simulink model "PMSM_lab"  (Simulink 10.0)
settings: Solver=ode4  StartTime=0.0  StopTime=2  FixedStep=1e-4  RelTol=1e-3  EnableMultiTasking=on
InitFcn:
  | Vdc=530;
  | P=8;
  | Rs=1.477;
  | Lds=19.75e-3;
  | Lqs=22.5e-3;
  | flux=0.2068;
  | J=0.0015806;
  | B=0.0034;
  | Wc=2*pi*500;
  | PM=75*pi/180;
  | Wc_kp_by_kids=tan(PM-pi/2+atan(Wc*Lds/Rs));
  | kids=Wc*sqrt(Rs*Rs+(Wc*Lds)^2)/sqrt(Wc_kp_by_kids^2+1);
  | kpds=Wc_kp_by_kids*kids/Wc;
  | Wc_kp_by_kiqs=tan(PM-pi/2+atan(Wc*Lqs/Rs));
  | kiqs=Wc*sqrt(Rs*Rs+(Wc*Lqs)^2)/sqrt(Wc_kp_by_kiqs^2+1);
  | kpqs=Wc_kp_by_kiqs*kiqs/Wc;
  | Wcw=2*pi*42;
  | PM=78*pi/180;
  | Wc_kp_by_kiw=tan(PM-pi/2+atan(Wcw*J/B));
  | kiw=(Wcw*sqrt(B*B+(Wcw*J)^2))/((3/2)*(P/2)*flux*sqrt(Wc_kp_by_kiw^2+1));
  | kpw=Wc_kp_by_kiw*kiw/Wcw;
  | 
  | 
  | PM  = 75;
  | Wc = 3140;
  | R=1.6;
  | Lq = 0.0225;
  | Ld = 0.01975;
  | 
  | PI_q = tand(PM - 90 + atand((Wc*Lq)/R));
  | Ki_q = (Wc * sqrt(((R)^2)+((Wc*Lq)^2))/sqrt(1+(PI_q)^2));
  | Kp_q = (PI_q * Ki_q)/Wc;
  | PI_d = tand(PM - 90 + atand((Wc*Ld)/R));
  | Ki_d = (Wc * sqrt(((R)^2)+((Wc*Ld)^2))/sqrt(1+(PI_d)^2));
  | Kp_d = (PI_d * Ki_d)/Wc;
  | 
  | 
  | Wc=2*pi*42;
  | PM=78;
  | wpi=tand(PM-90+atand((Wc*180/pi)*J/B));
  | Ki= (Wc * sqrt(B^2 + (Wc*J)^2))/(sqrt(1+(wpi)^2));
  | Kp= (wpi*Ki)/(Wc);
libraries: simulink x4, dsparch4 x3
settings Model: Creator=Gopi  LastModifiedBy=kanth
settings DataIOCC: LimitDataPoints=on  SignalLoggingSaveFormat=ModelDataLogs
settings OptimizationCC: ExpressionDepthLimit=2147483647
settings DebuggingCC: SolverPrmCheckMsg=warning  FcnCallInpInsideContextMsg=warning  StateNameClashWarn=warning
settings SFSimCC: SimParseCustomCode=off
settings GRTTargetCC: GeneratePreprocessorConditionals=Disable all
settings ConfigComp: CovExternalEMLEnable=off

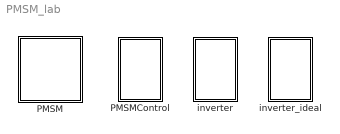
== system PMSM_lab ==
  PMSM : Subsystem
  PMSMControl : Subsystem
  inverter : Subsystem
  inverter_ideal : Subsystem

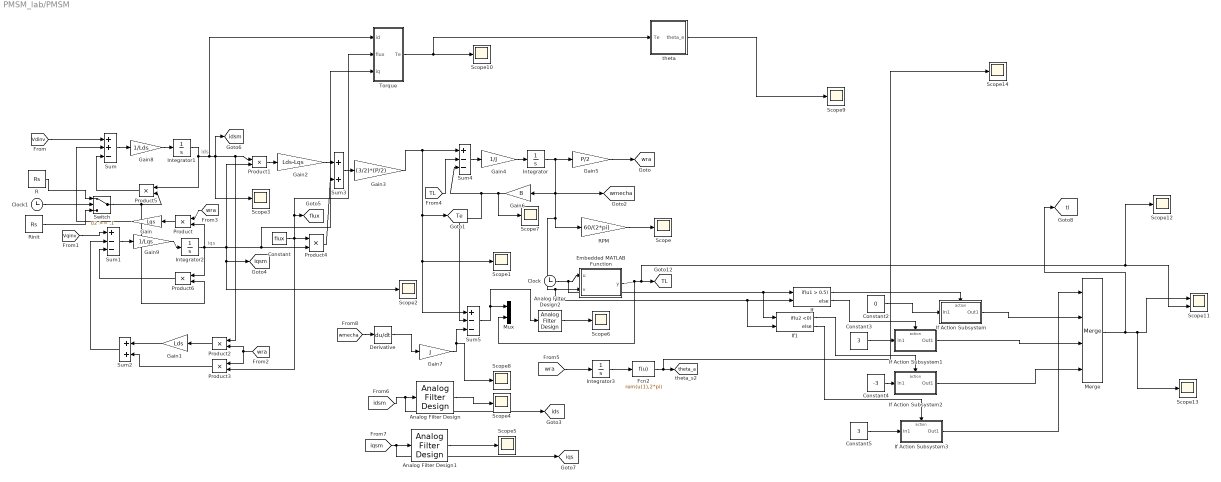
== system PMSM_lab/PMSM ==
  note: ids
  note: iqs
  Analog Filter Design : dsparch4/Analog Filter Design  method=Butterworth  filttype=Lowpass  N=1  Wlo=2*pi*1200  Whi=80  Rp=2  Rs=40
  Analog Filter Design1 : dsparch4/Analog Filter Design  method=Butterworth  filttype=Lowpass  N=1  Wlo=2*pi*800  Whi=80  Rp=2  Rs=40
  Analog Filter Design2 : dsparch4/Analog Filter Design  method=Butterworth  filttype=Lowpass  N=2  Wlo=2*pi*1000  Whi=80  Rp=2  Rs=40
  Clock : Clock
  Clock1 : Clock
  Constant : Constant  Value=flux
  Constant2 : Constant  Value=0
  Constant3 : Constant  Value=3
  Constant4 : Constant  Value=-3
  Constant5 : Constant  Value=3
  Derivative : Derivative
  Embedded MATLAB Function : MATLAB Function  TreatAsAtomicUnit=on
  Fcn2 : Fcn  Expr=rem(u(1),2*pi)
  Gain : Gain  Gain=Lqs
  Gain1 : Gain  Gain=Lds
  Gain2 : Gain  Gain=Lds-Lqs
  Gain3 : Gain  Gain=(3/2)*(P/2)
  Gain4 : Gain  Gain=1/J
  Gain5 : Gain  Gain=P/2
  Gain6 : Gain  Gain=B
  Gain7 : Gain  Gain=J
  Gain8 : Gain  Gain=1/Lds
  Gain9 : Gain  Gain=1/Lqs
  If : If  NumInputs=2  IfExpression=u1 > 0.5
  If Action Subsystem : Subsystem  TreatAsAtomicUnit=on
  If Action Subsystem1 : Subsystem  TreatAsAtomicUnit=on
  If Action Subsystem2 : Subsystem  TreatAsAtomicUnit=on
  If Action Subsystem3 : Subsystem  TreatAsAtomicUnit=on
  If1 : If  NumInputs=2  IfExpression=u2 <0
  Integrator{,1..3} (4 alike) : Integrator
  Merge : Merge  Inputs=4
  Mux : Mux  Inputs=2
  Product{,1..6} (7 alike) : Product  RndMeth=Zero
  R : Constant  Value=Rs
  RPM : Gain  Gain=60/(2*pi)
  Rinit : Constant  Value=Rs
  Scope{,1..10,12..14} (14 alike) : Scope
  Scope11 : Scope  NumInputPorts=2
  Sum : Sum  Inputs=++-
  Sum1 : Sum  Inputs=+--
  Sum2 : Sum
  Sum3 : Sum
  Sum4 : Sum  Inputs=+--
  Sum5 : Sum  Inputs=+--
  Switch : Switch  Threshold=.1
  Torque : Subsystem
  theta : Subsystem
  tag scope: TL=global, Te=global, flux=global, ids=global, idsm=global, iqs=global, iqsm=global, theta_a=global, tl=global, wmecha=global, wra=global
  wires:
  [Vdinv] -> Sum/1
  Gain/1 -> Sum/2
  Sum/1 -> Gain8/1
  Product/1 -> Gain/1
  Integrator1/1 -> Torque/1(id), Product1/1, Product2/1, Scope3/1, [idsm], Product5/1
  Sum1/1 -> Gain9/1
  Gain1/1 -> Sum2/1
  Sum2/1 -> Sum1/2
  Product2/1 -> Gain1/1
  Product3/1 -> Sum2/2
  Integrator2/1 -> [iqsm], Scope2/1, Product1/2, Torque/3(iq), Product4/2, Product/2, Product6/1
  Product1/1 -> Gain2/1
  Gain2/1 -> Sum3/1
  Product4/1 -> Sum3/2
  Sum3/1 -> Gain3/1
  [TL] -> Sum4/2
  Sum4/1 -> Gain4/1
  Gain4/1 -> Integrator/1
  [wra] -> Product/1
  Integrator/1 -> Gain5/1, [wmecha], RPM/1, If1/2, If/2, Embedded MATLAB Function/2(v), Gain6/1
  Gain5/1 -> [wra]
  Clock/1 -> If/1, If1/1, Embedded MATLAB Function/1(u)
  Embedded MATLAB Function/1(y) -> Scope12/1, Scope11/2, [TL], Mux/2
  RPM/1 -> Scope/1
  [Vqinv] -> Sum1/1
  Product5/1 -> Sum/3
  Product6/1 -> Sum1/3
  Gain8/1 -> Integrator1/1
  Gain9/1 -> Integrator2/1
  Clock1/1 -> Switch/2
  R/1 -> Switch/1
  Rinit/1 -> Switch/3
  Switch/1 -> Product5/2, Product6/2
  Integrator3/1 -> Fcn2/1
  [wra] -> Integrator3/1
  Fcn2/1 -> Scope14/1, [theta_a]
  Gain6/1 -> Sum4/3, Sum5/2, Scope7/1
  [wra] -> Product3/1, Product2/2
  [idsm] -> Analog Filter Design/1, [ids]
  [iqsm] -> Analog Filter Design1/1, [iqs]
  Analog Filter Design/1 -> Scope4/1
  Analog Filter Design1/1 -> Scope5/1
  [wmecha] -> Derivative/1
  Derivative/1 -> Gain7/1
  Gain7/1 -> Sum5/3, Scope8/1
  Sum5/1 -> Mux/1, Analog Filter Design2/1
  Analog Filter Design2/1 -> Scope6/1
  Constant/1 -> Torque/2(flux), [flux], Product3/2, Product4/1
  Torque/1(Te) -> theta/1(Te), Scope10/1
  Gain3/1 -> Sum4/1, [Te], Scope1/1, Sum5/1
  If/1 -> If Action Subsystem/Action
  Constant2/1 -> If Action Subsystem/1(In1)
  If/2 -> If Action Subsystem1/Action
  Constant3/1 -> If Action Subsystem1/1(In1)
  If Action Subsystem1/1(Out1) -> Merge/3
  If1/1 -> If Action Subsystem2/Action
  Constant4/1 -> If Action Subsystem2/1(In1)
  If Action Subsystem2/1(Out1) -> Merge/4
  If1/2 -> If Action Subsystem3/Action
  Constant5/1 -> If Action Subsystem3/1(In1)
  If Action Subsystem3/1(Out1) -> Merge/1
  If Action Subsystem/1(Out1) -> Merge/2
  Merge/1 -> [tl], Scope13/1, Scope11/1
  theta/1(theta_e) -> Scope9/1

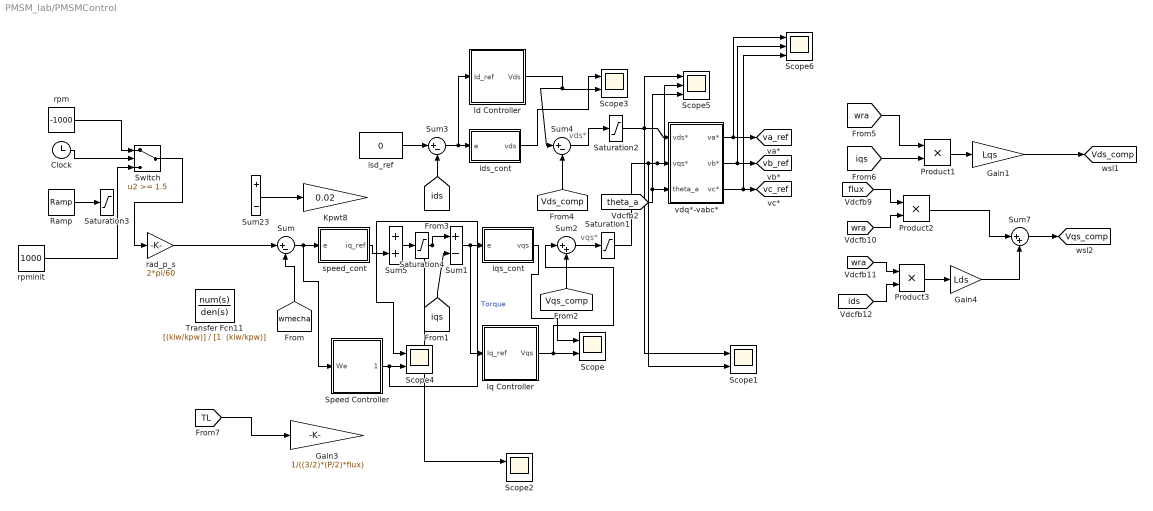
== system PMSM_lab/PMSMControl ==
  note: vds*
  note: vqs*
  Clock : Clock
  Gain1 : Gain  Gain=Lqs
  Gain3 : Gain  Gain=1/((3/2)*(P/2)*flux)
  Gain4 : Gain  Gain=Lds
  Id Controller : Subsystem
  Iq Controller : Subsystem
  Kpwt8 : Gain  Gain=0.02
  Product1 : Product  RndMeth=Zero
  Product2 : Product  RndMeth=Zero
  Product3 : Product  RndMeth=Zero
  Ramp : simulink/Sources/Ramp  slope=2000/(0.1)  start=0  InitialOutput=200
  Saturation1 : Saturate  UpperLimit=220  LowerLimit=-220
  Saturation2 : Saturate  UpperLimit=220  LowerLimit=-220
  Saturation3 : Saturate  UpperLimit=2000  LowerLimit=-2000
  Saturation4 : Saturate  UpperLimit=5  LowerLimit=-5
  Scope{,1..4} (5 alike) : Scope  NumInputPorts=2
  Scope5 : Scope  NumInputPorts=3
  Scope6 : Scope  NumInputPorts=3
  Speed Controller : Subsystem
  Sum : Sum  Inputs=|+-
  Sum1 : Sum  Inputs=+-
  Sum2 : Sum  Inputs=|++
  Sum23 : Sum  Inputs=+-
  Sum3 : Sum  Inputs=|+-
  Sum4 : Sum  Inputs=|+-
  Sum5 : Sum
  Sum7 : Sum  Inputs=|++
  Switch : Switch  Threshold=1.5
  Transfer Fcn11 : TransferFcn  Numerator=[(kiw/kpw)]  Denominator="[1  (kiw/kpw)]"
  ids_cont : Subsystem
  iqs_cont : Subsystem
  isd_ref : Constant  Value=0
  rad_p_s : Gain  Gain=2*pi/60
  rpm : Constant  Value=-1000
  rpminit : Constant  Value=1000
  speed_cont : Subsystem
  vdq*-vabc* : Subsystem
  tag scope: Vds_comp=global, Vqs_comp=global, va_ref=global, vb_ref=global, vc_ref=global
  wires:
  [wmecha] -> Sum/2
  Sum/1 -> Speed Controller/1(We), speed_cont/1(e)
  Sum1/1 -> Iq Controller/1(Iq_ref), iqs_cont/1(e)
  iqs_cont/1(vqs) -> Scope/1
  [Vqs_comp] -> Sum2/2
  isd_ref/1 -> Sum3/1
  [ids] -> Sum3/2
  Sum3/1 -> Id Controller/1(Id_ref), ids_cont/1(e)
  ids_cont/1(vds) -> Scope3/1
  [Vds_comp] -> Sum4/2
  Sum2/1 -> Saturation1/1
  Sum4/1 -> Saturation2/1
  [theta_a] -> Scope5/3, vdq*-vabc*/3(theta_a)
  vdq*-vabc*/1(va*) -> Scope6/1, [va_ref]
  vdq*-vabc*/2(vb*) -> Scope6/2, [vb_ref]
  vdq*-vabc*/3(vc*) -> Scope6/3, [vc_ref]
  [flux] -> Product2/1
  [wra] -> Product2/2
  Product2/1 -> Sum7/1
  [wra] -> Product3/1
  [ids] -> Product3/2
  Product3/1 -> Gain4/1
  Gain4/1 -> Sum7/2
  Sum7/1 -> [Vqs_comp]
  [wra] -> Product1/1
  [iqs] -> Product1/2
  Product1/1 -> Gain1/1
  Gain1/1 -> [Vds_comp]
  rad_p_s/1 -> Sum/1
  Clock/1 -> Switch/2
  rpm/1 -> Switch/1
  Switch/1 -> rad_p_s/1
  Saturation2/1 -> Scope5/1, vdq*-vabc*/1(vds*), Scope1/1
  Saturation1/1 -> Scope5/2, vdq*-vabc*/2(vqs*), Scope1/2
  Ramp/1 -> Saturation3/1
  rpminit/1 -> Switch/3
  Sum23/1 -> Kpwt8/1
  [iqs] -> Sum1/2
  speed_cont/1(iq_ref) -> Scope4/1
  Sum5/1 -> Saturation4/1
  Saturation4/1 -> Sum1/1, Scope2/1
  [TL] -> Gain3/1
  Iq Controller/1(Vqs) -> Sum2/1, Scope/2
  Id Controller/1(Vds) -> Sum4/1, Scope3/2
  Speed Controller/1(Torque) -> Sum5/2, Scope4/2  "Torque"

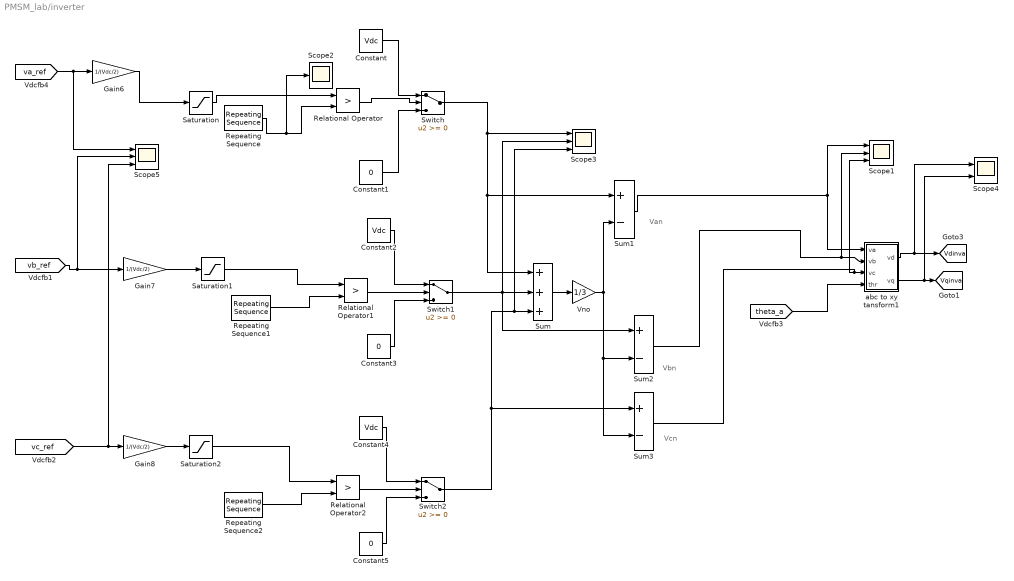
== system PMSM_lab/inverter ==
  note: Vbn
  note: Vcn
  note: Van
  Constant : Constant  Value=Vdc
  Constant1 : Constant  Value=0
  Constant2 : Constant  Value=Vdc
  Constant3 : Constant  Value=0
  Constant4 : Constant  Value=Vdc
  Constant5 : Constant  Value=0
  Gain6 : Gain  Gain=1/(Vdc/2)
  Gain7 : Gain  Gain=1/(Vdc/2)
  Gain8 : Gain  Gain=1/(Vdc/2)
  Relational Operator : RelationalOperator  Operator=>  OutDataTypeStr=boolean  RndMeth=Nearest
  Relational Operator1 : RelationalOperator  Operator=>  OutDataTypeStr=boolean  RndMeth=Nearest
  Relational Operator2 : RelationalOperator  Operator=>  OutDataTypeStr=boolean  RndMeth=Nearest
  Repeating Sequence : simulink/Sources/Repeating Sequence  rep_seq_t=[0 1/(2*5000) 1/5000]  rep_seq_y=[-1 1 -1]
  Repeating Sequence1 : simulink/Sources/Repeating Sequence  rep_seq_t=[0 1/(2*5000) 1/5000]  rep_seq_y=[-1 1 -1]
  Repeating Sequence2 : simulink/Sources/Repeating Sequence  rep_seq_t=[0 1/(2*5000) 1/5000]  rep_seq_y=[-1 1 -1]
  Saturation : Saturate  UpperLimit=0.9  LowerLimit=-0.9
  Saturation1 : Saturate  UpperLimit=0.9  LowerLimit=-0.9
  Saturation2 : Saturate  UpperLimit=0.9  LowerLimit=-0.9
  Scope1 : Scope  NumInputPorts=3
  Scope2 : Scope
  Scope3 : Scope  NumInputPorts=3
  Scope4 : Scope  NumInputPorts=2
  Scope5 : Scope  NumInputPorts=3
  Sum : Sum  Inputs=+++
  Sum1 : Sum  Inputs=+-
  Sum2 : Sum  Inputs=+-
  Sum3 : Sum  Inputs=+-
  Switch : Switch
  Switch1 : Switch
  Switch2 : Switch
  Vno : Gain  Gain=1/3
  abc to xy tansform1 : Subsystem
  tag scope: Vdinva=global, Vqinva=global
  wires:
  Gain6/1 -> Saturation/1
  Repeating Sequence/1 -> Relational Operator/2, Scope2/1
  Relational Operator/1 -> Switch/2
  Constant/1 -> Switch/1
  Constant1/1 -> Switch/3
  Repeating Sequence1/1 -> Relational Operator1/2
  Relational Operator1/1 -> Switch1/2
  Constant2/1 -> Switch1/1
  Constant3/1 -> Switch1/3
  Gain8/1 -> Saturation2/1
  Repeating Sequence2/1 -> Relational Operator2/2
  Relational Operator2/1 -> Switch2/2
  Constant4/1 -> Switch2/1
  Constant5/1 -> Switch2/3
  Switch/1 -> Scope3/1, Sum/1, Sum1/1
  Switch1/1 -> Scope3/2, Sum2/1, Sum/2
  Switch2/1 -> Scope3/3, Sum/3, Sum3/1
  Sum/1 -> Vno/1
  Vno/1 -> Sum1/2, Sum2/2, Sum3/2
  [va_ref] -> Scope5/1, Gain6/1
  [vb_ref] -> Scope5/2, Gain7/1
  Gain7/1 -> Saturation1/1
  [vc_ref] -> Scope5/3, Gain8/1
  [theta_a] -> abc to xy tansform1/4(thr)
  abc to xy tansform1/1(vd) -> Scope4/1, [Vdinva]
  abc to xy tansform1/2(vq) -> Scope4/2, [Vqinva]
  Sum1/1 -> Scope1/1, abc to xy tansform1/1(va)
  Sum2/1 -> Scope1/2, abc to xy tansform1/2(vb)
  Sum3/1 -> Scope1/3, abc to xy tansform1/3(vc)
  Saturation/1 -> Relational Operator/1
  Saturation1/1 -> Relational Operator1/1
  Saturation2/1 -> Relational Operator2/1

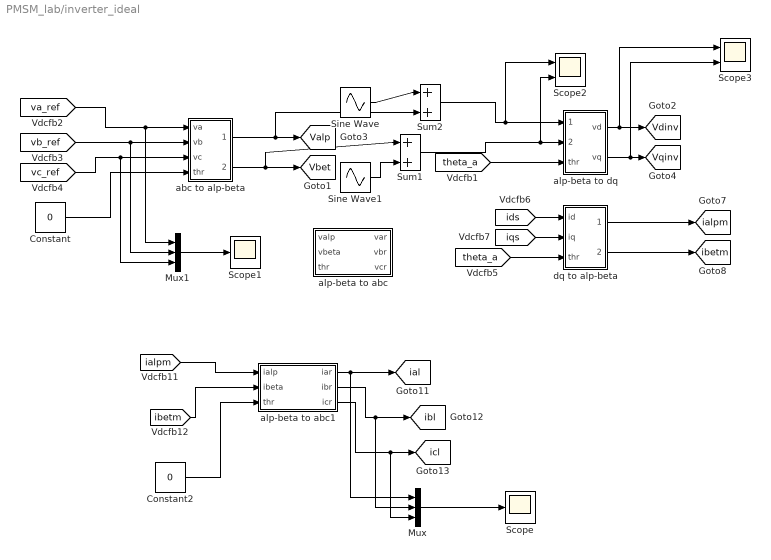
== system PMSM_lab/inverter_ideal ==
  Constant : Constant  Value=0
  Constant2 : Constant  Value=0
  Mux : Mux  Inputs=3
  Mux1 : Mux  Inputs=3
  Scope : Scope
  Scope1 : Scope
  Scope2 : Scope  NumInputPorts=2
  Scope3 : Scope  NumInputPorts=2
  Sine Wave : Sin  Amplitude=0  Frequency=2*pi*1000  SampleTime=0
  Sine Wave1 : Sin  Amplitude=0  Frequency=2*pi*1000  Phase=pi/2  SampleTime=0
  Sum1 : Sum  Inputs=|++
  Sum2 : Sum  Inputs=|++
  abc to alp-beta : Subsystem
  alp-beta to abc : Subsystem
  alp-beta to abc1 : Subsystem
  alp-beta to dq : Subsystem
  dq to alp-beta : Subsystem
  tag scope: Valp=global, Vbet=global, Vdinv=global, Vqinv=global, ial=global, ialpm=global, ibetm=global, ibl=global, icl=global
  wires:
  abc to alp-beta/2(vbeta) -> [Vbet], Sum1/1
  abc to alp-beta/1(valp) -> [Valp], Sum2/2
  Constant/1 -> abc to alp-beta/4(thr)
  [vb_ref] -> abc to alp-beta/2(vb), Mux1/2
  [va_ref] -> abc to alp-beta/1(va), Mux1/1
  [vc_ref] -> abc to alp-beta/3(vc), Mux1/3
  [theta_a] -> alp-beta to dq/3(thr)
  [theta_a] -> dq to alp-beta/3(thr)
  alp-beta to dq/1(vd) -> Scope3/1, [Vdinv]
  alp-beta to dq/2(vq) -> Scope3/2, [Vqinv]
  [ids] -> dq to alp-beta/1(id)
  [iqs] -> dq to alp-beta/2(iq)
  dq to alp-beta/1(ialp) -> [ialpm]
  dq to alp-beta/2(ibet) -> [ibetm]
  Sine Wave/1 -> Sum2/1
  Sum2/1 -> Scope2/1, alp-beta to dq/1(valp)
  Sine Wave1/1 -> Sum1/2
  Sum1/1 -> Scope2/2, alp-beta to dq/2(vbet)
  [ialpm] -> alp-beta to abc1/1(ialp)
  [ibetm] -> alp-beta to abc1/2(ibeta)
  Constant2/1 -> alp-beta to abc1/3(thr)
  alp-beta to abc1/1(iar) -> [ial], Mux/1
  alp-beta to abc1/2(ibr) -> [ibl], Mux/2
  alp-beta to abc1/3(icr) -> [icl], Mux/3
  Mux/1 -> Scope/1
  Mux1/1 -> Scope1/1

== system PMSM_lab/PMSM/If Action Subsystem ==
  In1 : Inport
  Action Port : ActionPort  ActionPortLabel=if(u1 > 0.5)
  Out1 : Outport
  wires:
  In1/1 -> Out1/1

== system PMSM_lab/PMSM/If Action Subsystem1 ==
  In1 : Inport
  Action Port : ActionPort  ActionPortLabel=else
  Out1 : Outport
  wires:
  In1/1 -> Out1/1

== system PMSM_lab/PMSM/If Action Subsystem2 ==
  In1 : Inport
  Action Port : ActionPort  ActionPortLabel=if(u2 <0)
  Out1 : Outport
  wires:
  In1/1 -> Out1/1

== system PMSM_lab/PMSM/If Action Subsystem3 ==
  In1 : Inport
  Action Port : ActionPort  ActionPortLabel=else
  Out1 : Outport
  wires:
  In1/1 -> Out1/1

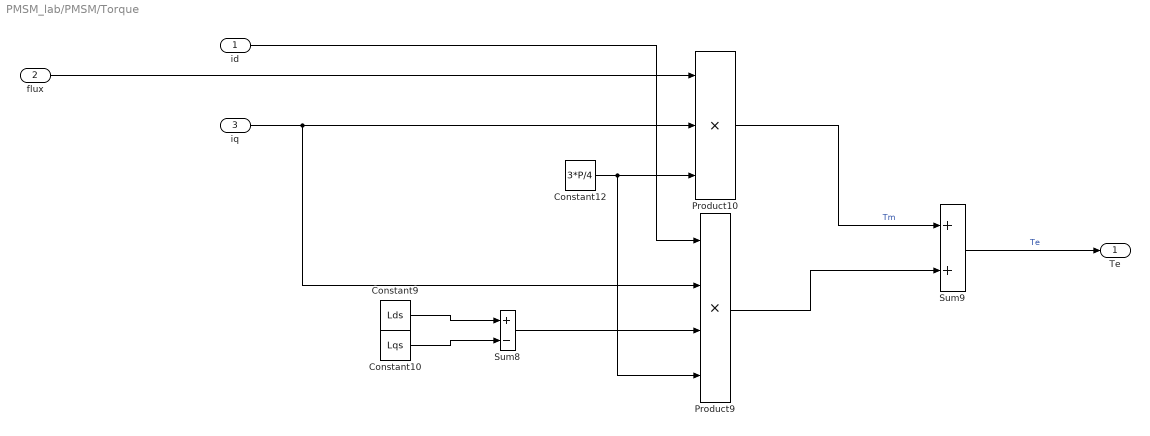
== system PMSM_lab/PMSM/Torque ==
  id : Inport
  flux : Inport  Port=2
  iq : Inport  Port=3
  Constant10 : Constant  Value=Lqs
  Constant12 : Constant  Value=3*P/4
  Constant9 : Constant  Value=Lds
  Product10 : Product  Inputs=3
  Product9 : Product  Inputs=4
  Sum8 : Sum  Inputs=+-
  Sum9 : Sum
  Te : Outport
  wires:
  id/1 -> Product9/1
  iq/1 -> Product9/2, Product10/2
  flux/1 -> Product10/1
  Constant12/1 -> Product9/4, Product10/3
  Product9/1 -> Sum9/2
  Sum8/1 -> Product9/3
  Constant10/1 -> Sum8/2
  Product10/1 -> Sum9/1  "Tm"
  Constant9/1 -> Sum8/1
  Sum9/1 -> Te/1  "Te"

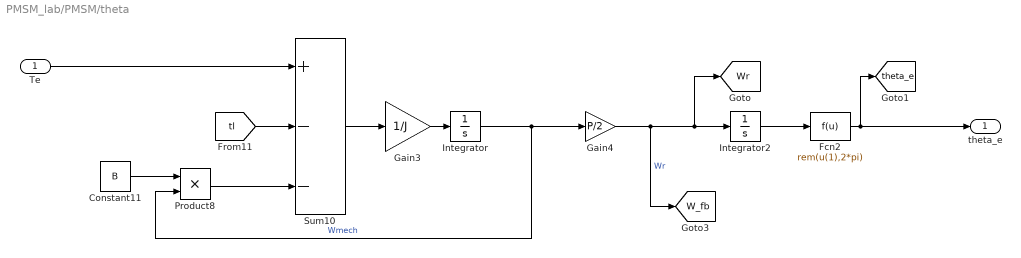
== system PMSM_lab/PMSM/theta ==
  Te : Inport
  Constant11 : Constant  Value=B
  Fcn2 : Fcn  Expr=rem(u(1),2*pi)
  Gain3 : Gain  Gain=1/J
  Gain4 : Gain  Gain=P/2
  Integrator : Integrator
  Integrator2 : Integrator
  Product8 : Product
  Sum10 : Sum  Inputs=+--
  theta_e : Outport
  tag scope: W_fb=global, Wr=global, theta_e=global
  wires:
  Sum10/1 -> Gain3/1
  Gain3/1 -> Integrator/1
  Product8/1 -> Sum10/3
  Integrator2/1 -> Fcn2/1
  Fcn2/1 -> theta_e/1, [theta_e]
  Constant11/1 -> Product8/1
  Gain4/1 -> [W_fb], Integrator2/1, [Wr]  "Wr"
  [tl] -> Sum10/2
  Te/1 -> Sum10/1
  Integrator/1 -> Product8/2, Gain4/1  "Wmech"

== system PMSM_lab/PMSMControl/Id Controller ==
  Id_ref : Inport
  "  1" : Gain  Gain=Ki_d
  " 1" : Gain  Gain=Kp_d
  Integrator1 : Integrator  LimitOutput=on  UpperSaturationLimit=200  LowerSaturationLimit=-200
  Saturation1 : Saturate  UpperLimit=220  LowerLimit=-220
  Sum5 : Sum  Inputs=|++
  Vds : Outport
  wires:
  "  1"/1 -> Integrator1/1
  Id_ref/1 -> " 1"/1, "  1"/1
  Integrator1/1 -> Sum5/2
  Sum5/1 -> Saturation1/1
  Saturation1/1 -> Vds/1
  " 1"/1 -> Sum5/1

== system PMSM_lab/PMSMControl/Iq Controller ==
  Iq_ref : Inport
  " " : Gain  Gain=Kp_q
  "  " : Gain  Gain=Ki_q
  Integrator : Integrator  LimitOutput=on  UpperSaturationLimit=200  LowerSaturationLimit=-200
  Saturation : Saturate  UpperLimit=220  LowerLimit=-220
  Sum2 : Sum  Inputs=|++
  Vqs : Outport
  wires:
  "  "/1 -> Integrator/1
  Sum2/1 -> Saturation/1
  " "/1 -> Sum2/1
  Integrator/1 -> Sum2/2
  Iq_ref/1 -> "  "/1, " "/1
  Saturation/1 -> Vqs/1  "Voltage"

== system PMSM_lab/PMSMControl/Speed Controller ==
  We : Inport
  " " : Gain  Gain=Kp
  "  " : Gain  Gain=Ki
  Gain : Gain  Gain=4/(3*P*flux)
  Integrator : Integrator  LimitOutput=on  UpperSaturationLimit=4.5  LowerSaturationLimit=-4.5
  Saturation : Saturate  UpperLimit=5  LowerLimit=-5
  Sum1 : Sum  Inputs=|++
  Torque : Outport
  wires:
  We/1 -> "  "/1, " "/1
  " "/1 -> Sum1/1
  Integrator/1 -> Sum1/2
  "  "/1 -> Integrator/1
  Saturation/1 -> Gain/1
  Sum1/1 -> Saturation/1
  Gain/1 -> Torque/1  "Current (Iq_ref)"

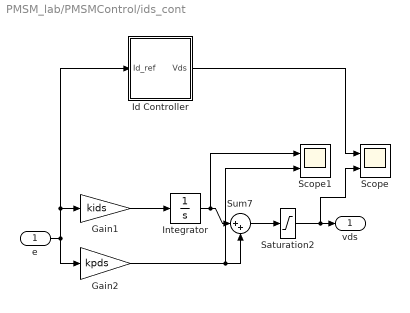
== system PMSM_lab/PMSMControl/ids_cont ==
  e : Inport
  Gain1 : Gain  Gain=kids
  Gain2 : Gain  Gain=kpds
  Id Controller : Subsystem
  Integrator : Integrator  LimitOutput=on  UpperSaturationLimit=200  LowerSaturationLimit=-200
  Saturation2 : Saturate  UpperLimit=220  LowerLimit=-220
  Scope : Scope  NumInputPorts=2
  Scope1 : Scope  NumInputPorts=2
  Sum7 : Sum  Inputs=|++
  vds : Outport
  wires:
  Gain1/1 -> Integrator/1
  Integrator/1 -> Sum7/1, Scope1/1
  Gain2/1 -> Sum7/2, Scope1/2
  e/1 -> Id Controller/1(Id_ref), Gain1/1, Gain2/1
  Sum7/1 -> Saturation2/1
  Saturation2/1 -> Scope/2, vds/1
  Id Controller/1(Vds) -> Scope/1

== system PMSM_lab/PMSMControl/iqs_cont ==
  e : Inport
  Gain1 : Gain  Gain=kiqs
  Gain2 : Gain  Gain=kpqs
  Integrator : Integrator  LimitOutput=on  UpperSaturationLimit=200  LowerSaturationLimit=-200
  Saturation2 : Saturate  UpperLimit=220  LowerLimit=-220
  Scope1 : Scope  NumInputPorts=2
  Sum7 : Sum  Inputs=|++
  Unit Delay3 : UnitDelay  SampleTime=-1
  vqs : Outport
  wires:
  Gain1/1 -> Integrator/1
  Integrator/1 -> Sum7/1, Scope1/1
  Gain2/1 -> Sum7/2, Scope1/2
  e/1 -> Gain1/1, Gain2/1
  Sum7/1 -> Saturation2/1
  Unit Delay3/1 -> vqs/1
  Saturation2/1 -> Unit Delay3/1

== system PMSM_lab/PMSMControl/speed_cont ==
  e : Inport
  Gain1 : Gain  Gain=kiw
  Gain2 : Gain  Gain=kpw
  Integrator : Integrator  LimitOutput=on  UpperSaturationLimit=4.5  LowerSaturationLimit=-4.5
  Saturation1 : Saturate  UpperLimit=5  LowerLimit=-5
  Sum7 : Sum  Inputs=|++
  iq_ref : Outport
  wires:
  Integrator/1 -> Sum7/1
  Gain2/1 -> Sum7/2
  e/1 -> Gain1/1, Gain2/1
  Sum7/1 -> Saturation1/1
  Saturation1/1 -> iq_ref/1
  Gain1/1 -> Integrator/1  "Current (Iq_ref)"

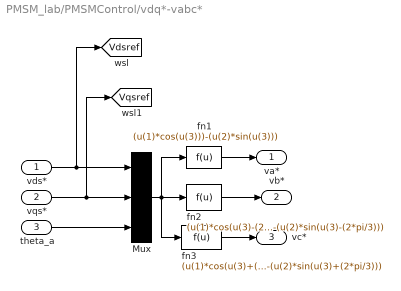
== system PMSM_lab/PMSMControl/vdq*-vabc* ==
  vds* : Inport
  vqs* : Inport  Port=2
  theta_a : Inport  Port=3
  Mux : Mux  Inputs=3
  fn1 : Fcn  Expr=(u(1)*cos(u(3)))-(u(2)*sin(u(3)))
  fn2 : Fcn  Expr=(u(1)*cos(u(3)-(2*pi/3)))-(u(2)*sin(u(3)-(2*pi/3)))
  fn3 : Fcn  Expr=(u(1)*cos(u(3)+(2*pi/3)))-(u(2)*sin(u(3)+(2*pi/3)))
  va* : Outport
  vb* : Outport  Port=2
  vc* : Outport  Port=3
  tag scope: Vdsref=global, Vqsref=global
  wires:
  Mux/1 -> fn1/1, fn3/1, fn2/1
  theta_a/1 -> Mux/3
  vqs*/1 -> Mux/2, [Vqsref]
  vds*/1 -> Mux/1, [Vdsref]
  fn3/1 -> vc*/1
  fn2/1 -> vb*/1
  fn1/1 -> va*/1

== system PMSM_lab/inverter/abc to xy tansform1 ==
  va : Inport
  vb : Inport  Port=2
  vc : Inport  Port=3
  thr : Inport  Port=4
  Fcn : Fcn  Expr=((u(1)*cos(u(4)))+(u(2)*cos(u(4)-2*pi/3))+(u(3)*cos(u(4)+(2*pi/3))))*(2/3)
  Fcn1 : Fcn  Expr=-((u(1)*sin(u(4)))+(u(2)*sin(u(4)-(2*pi/3)))+(u(3)*sin(u(4)+(2*pi/3))))*(2/3)
  Mux : Mux
  vd : Outport
  vq : Outport  Port=2
  wires:
  vb/1 -> Mux/2
  vc/1 -> Mux/3
  thr/1 -> Mux/4
  va/1 -> Mux/1
  Mux/1 -> Fcn/1, Fcn1/1
  Fcn/1 -> vd/1
  Fcn1/1 -> vq/1

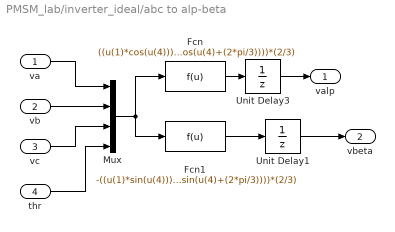
== system PMSM_lab/inverter_ideal/abc to alp-beta ==
  va : Inport
  vb : Inport  Port=2
  vc : Inport  Port=3
  thr : Inport  Port=4
  Fcn : Fcn  Expr=((u(1)*cos(u(4)))+(u(2)*cos(u(4)-2*pi/3))+(u(3)*cos(u(4)+(2*pi/3))))*(2/3)
  Fcn1 : Fcn  Expr=-((u(1)*sin(u(4)))+(u(2)*sin(u(4)-(2*pi/3)))+(u(3)*sin(u(4)+(2*pi/3))))*(2/3)
  Mux : Mux
  Unit Delay1 : UnitDelay  SampleTime=-1
  Unit Delay3 : UnitDelay  SampleTime=-1
  valp : Outport
  vbeta : Outport  Port=2
  wires:
  Fcn1/1 -> Unit Delay1/1
  Fcn/1 -> Unit Delay3/1
  Mux/1 -> Fcn1/1, Fcn/1
  va/1 -> Mux/1
  thr/1 -> Mux/4
  vc/1 -> Mux/3
  vb/1 -> Mux/2
  Unit Delay3/1 -> valp/1
  Unit Delay1/1 -> vbeta/1

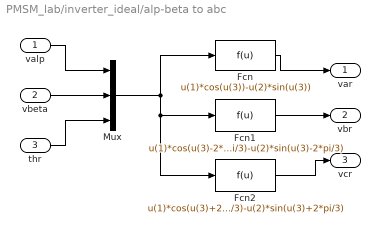
== system PMSM_lab/inverter_ideal/alp-beta to abc ==
  valp : Inport
  vbeta : Inport  Port=2
  thr : Inport  Port=3
  Fcn : Fcn  Expr=u(1)*cos(u(3))-u(2)*sin(u(3))
  Fcn1 : Fcn  Expr=u(1)*cos(u(3)-2*pi/3)-u(2)*sin(u(3)-2*pi/3)
  Fcn2 : Fcn  Expr=u(1)*cos(u(3)+2*pi/3)-u(2)*sin(u(3)+2*pi/3)
  Mux : Mux  Inputs=3
  var : Outport
  vbr : Outport  Port=2
  vcr : Outport  Port=3
  wires:
  valp/1 -> Mux/1
  vbeta/1 -> Mux/2
  thr/1 -> Mux/3
  Mux/1 -> Fcn/1, Fcn1/1, Fcn2/1
  Fcn/1 -> var/1
  Fcn1/1 -> vbr/1
  Fcn2/1 -> vcr/1

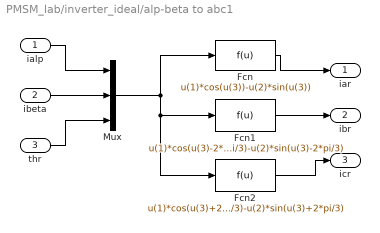
== system PMSM_lab/inverter_ideal/alp-beta to abc1 ==
  ialp : Inport
  ibeta : Inport  Port=2
  thr : Inport  Port=3
  Fcn : Fcn  Expr=u(1)*cos(u(3))-u(2)*sin(u(3))
  Fcn1 : Fcn  Expr=u(1)*cos(u(3)-2*pi/3)-u(2)*sin(u(3)-2*pi/3)
  Fcn2 : Fcn  Expr=u(1)*cos(u(3)+2*pi/3)-u(2)*sin(u(3)+2*pi/3)
  Mux : Mux  Inputs=3
  iar : Outport
  ibr : Outport  Port=2
  icr : Outport  Port=3
  wires:
  Fcn2/1 -> icr/1
  Fcn1/1 -> ibr/1
  Fcn/1 -> iar/1
  Mux/1 -> Fcn2/1, Fcn1/1, Fcn/1
  thr/1 -> Mux/3
  ibeta/1 -> Mux/2
  ialp/1 -> Mux/1

== system PMSM_lab/inverter_ideal/alp-beta to dq ==
  valp : Inport
  vbet : Inport  Port=2
  thr : Inport  Port=3
  Fcn : Fcn  Expr=(u(1)*cos(u(3)))+(u(2)*sin(u(3)))
  Fcn1 : Fcn  Expr=-(u(1)*sin(u(3)))+(u(2)*cos(u(3)))
  Mux : Mux  Inputs=3
  vd : Outport
  vq : Outport  Port=2
  wires:
  vbet/1 -> Mux/2
  thr/1 -> Mux/3
  valp/1 -> Mux/1
  Mux/1 -> Fcn/1, Fcn1/1
  Fcn/1 -> vd/1
  Fcn1/1 -> vq/1

== system PMSM_lab/inverter_ideal/dq to alp-beta ==
  id : Inport
  iq : Inport  Port=2
  thr : Inport  Port=3
  Fcn : Fcn  Expr=(u(1)*cos(u(3)))-(u(2)*sin(u(3)))
  Fcn1 : Fcn  Expr=(u(1)*sin(u(3)))+(u(2)*cos(u(3)))
  Mux : Mux  Inputs=3
  ialp : Outport
  ibet : Outport  Port=2
  wires:
  Fcn1/1 -> ibet/1
  Fcn/1 -> ialp/1
  Mux/1 -> Fcn1/1, Fcn/1
  id/1 -> Mux/1
  thr/1 -> Mux/3
  iq/1 -> Mux/2

== system PMSM_lab/PMSMControl/ids_cont/Id Controller ==
  Id_ref : Inport
  "  1" : Gain  Gain=Ki_d
  " 1" : Gain  Gain=Kp_d
  Integrator1 : Integrator  LimitOutput=on  UpperSaturationLimit=200  LowerSaturationLimit=-200
  Saturation1 : Saturate  UpperLimit=220  LowerLimit=-220
  Sum5 : Sum  Inputs=|++
  Vds : Outport
  wires:
  "  1"/1 -> Integrator1/1
  Id_ref/1 -> " 1"/1, "  1"/1
  Integrator1/1 -> Sum5/2
  Sum5/1 -> Saturation1/1
  Saturation1/1 -> Vds/1
  " 1"/1 -> Sum5/1

== matlab function PMSM/Embedded MATLAB Function ==
  data: u input double; y output double; v input double
function y = fcn(u,v)
%#eml
y=3;
if u>0.5
    y=0;
end
if v<0
    y=-y;
end
